simulink model "lab1_1"  (R2020b)
settings: Solver=VariableStepAuto  StartTime=0.0  StopTime=1  RelTol=1e-3
settings Model: Creator=Dexp  LastModifiedBy=takem

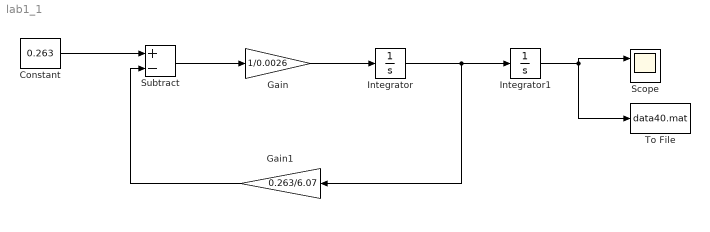
== system lab1_1 ==
  Constant : Constant  Value=0.263
  Gain : Gain  Gain=1/0.0026
  Gain1 : Gain  Gain=0.263/6.07
  Integrator : Integrator
  Integrator1 : Integrator
  Scope : Scope  NumInputPorts=2
  Subtract : Sum  Inputs=+-
  To File : ToFile  Filename=data40.mat  MatrixName=data
  wires:
  Constant/1 -> Subtract/1
  Subtract/1 -> Gain/1
  Gain/1 -> Integrator/1
  Integrator/1 -> Gain1/1, Integrator1/1
  Integrator1/1 -> To File/1, Scope/1
  Gain1/1 -> Subtract/2
